simulink model "SimulacaocomVTeCA"  (R2024b)
settings: Solver=VariableStepAuto  StartTime=0.0  StopTime=10  RelTol=1e-3
values from neighbouring files (symbols this model uses):
  AirTemperature = 303    [CodigoVT.m]
  C1 = 1.2801    [CodigoVT.m]
  C2 = 23.99    [CodigoVT.m]
  C3 = 0.52    [CodigoVT.m]
  VelRef = 30    [CodigoVT.m]
undefined symbols (not defined in the file or in its folder): EV, fractalcoef, MTR
libraries: vehdynlibtire x4, slpidlib x2, autolibmappedmotor x2, vrlib x1, mspsensorlib x1, vehdynlibviscommon x1, vehdynlibscenariocommon x1, vehdynlibsuspension x1, vehdynlibsteering x1, vehdynlibdriver x1, autolibshared x1
(part 3 of 3)

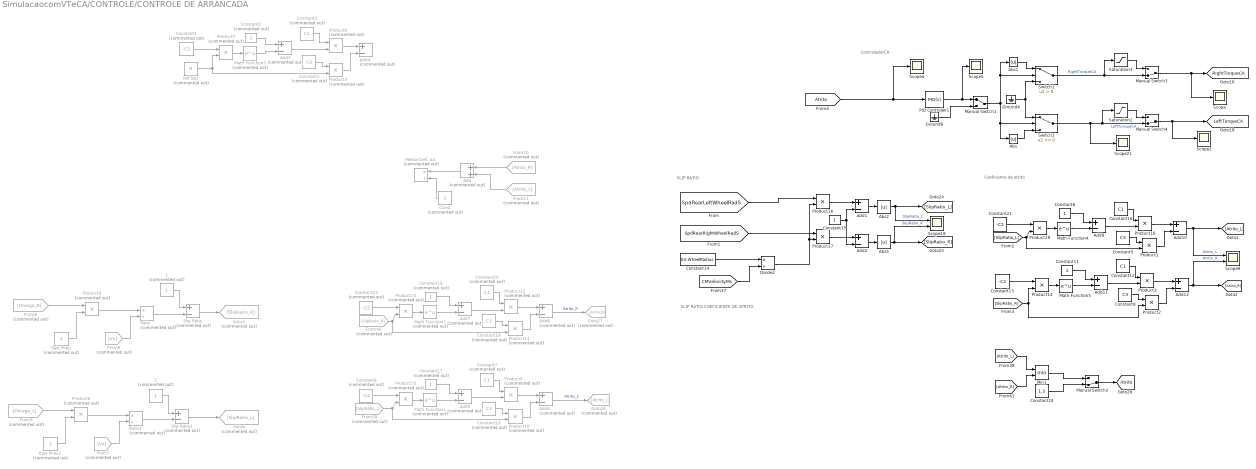
== system SimulacaocomVTeCA/CONTROLE/CONTROLE DE ARRANCADA  ==
  note: ControladorCA
  note: SLIP RATIO
  note: SLIP RATIO
      |
      | COEFICIENTE DE ATRITO
  note: Coeficiente de atrito
  1 : Constant  Commented=on
  2 : Constant  Commented=on
  Abs{,1..2,5} (4 alike) : Abs  SaturateOnIntegerOverflow=off
  Add : Sum  Commented=on
  Add{1..2,9..12} (6 alike) : Sum  Inputs=+-
  Add{3..8} (6 alike) : Sum  Commented=on  Inputs=+-
  Const : Constant  Commented=on  Value=2
  Constant1 : Constant  Commented=on  Value=C3
  Constant10 : Constant  Commented=on  Value=C3
  Constant11 : Constant
  Constant12 : Constant  Value=C1
  Constant13 : Constant  Value=-C2
  Constant14 : Constant  Value=EV.WheelRadius  VectorParams1D=off
  Constant15 : Constant
  Constant16 : Constant  Value=C1
  Constant17 : Constant  Commented=on
  Constant18 : Constant  Commented=on  Value=C3
  Constant19 : Constant  Commented=on
  Constant2 : Constant  Commented=on
  Constant20 : Constant  Commented=on  Value=C1
  Constant21 : Constant  Value=-C2
  Constant23 : Constant  Commented=on  Value=-C2
  Constant24 : Constant  Value=1.3  VectorParams1D=off
  Constant3 : Constant  Commented=on  Value=C1
  Constant4 : Constant  Commented=on  Value=-C2
  Constant5 : Constant  Value=C3
  Constant6 : Constant
  Constant7 : Constant  Commented=on  Value=C1
  Constant8 : Constant  Commented=on  Value=-C2
  Constant9 : Constant  Value=C3
  Divide2 : Product  Inputs=*/
  From10 : From  Commented=on  GotoTag=Atrito_R
  From11 : From  Commented=on  GotoTag=Atrito_L
  From39 : From  Commented=on  GotoTag=SlipRatio_L
  From40 : From  Commented=on  GotoTag=SlipRatio_R
  From6 : From  Commented=on  GotoTag=Vx
  From7 : From  Commented=on  GotoTag=Vx
  From8 : From  Commented=on  GotoTag=Omega_R
  From9 : From  Commented=on  GotoTag=Omega_L
  Goto26 : Goto  Commented=on  GotoTag=Atrito_L
  Goto27 : Goto  Commented=on  GotoTag=Atrito_R
  Goto3 : Goto  Commented=on  GotoTag=SlipRatio_R
  Goto6 : Goto  Commented=on  GotoTag=SlipRatio_L
  Ground4 : Ground
  Ground6 : Ground
  Manual Switch1 : ManualSwitch
  Manual Switch2 : ManualSwitch  CurrentSetting=0
  Manual Switch3 : ManualSwitch  CurrentSetting=0
  Manual Switch4 : ManualSwitch  CurrentSetting=0
  Math Function1 : Math  Commented=on
  Math Function2 : Math  Commented=on
  Math Function3 : Math  Commented=on
  Math Function4 : Math
  Math Function5 : Math
  Min1 : MinMax  Inputs=2
  Média Coef. Ad. : Product  Commented=on  Inputs=*/
  PID Controller1 : slpidlib/PID Controller  Controller=PID  Form=Parallel  TimeDomain=Continuous-time  UseExternalTs=off  SampleTime=-1  IntegratorMethod=Forward Euler  FilterMethod=Forward Euler  ControllerParametersSource=internal  P=1  I=1  UseKiTs=off  D=0  UseExternalDerivativeSource=off  N=100  UseFilter=on  TunerSelectOption=Transfer Function Based (PID Tuner App)  InitialConditionSource=internal  InitialConditionForIntegrator=0  InitialConditionForFilter=0  DifferentiatorICPrevScaledInput=0  ExternalReset=none  TrackingMode=off  Kt=1  LimitOutput=off  SatLimitsSource=internal  UpperSaturationLimit=inf  LowerSaturationLimit=-inf  LinearizeAsGain=on  AntiWindupMode=none  Kb=1  LimitIntegrator=off  UpperIntegratorSaturationLimit=inf  LowerIntegratorSaturationLimit=-inf  POutMin=[]  POutMax=[]  IOutMin=[]  IOutMax=[]  DOutMin=[]  DOutMax=[]  NOutMin=[]  NOutMax=[]  SumOutMin=[]  SumOutMax=[]  SaturationOutMin=[]  SaturationOutMax=[]  PParamMin=[]  PParamMax=[]  IParamMin=[]  IParamMax=[]  DParamMin=[]  DParamMax=[]  NParamMin=[]  NParamMax=[]  KbParamMin=[]  KbParamMax=[]  KtParamMin=[]  KtParamMax=[]  KbOutMin=[]  KbOutMax=[]  KtOutMin=[]  KtOutMax=[]  IntegratorOutMin=[]  IntegratorOutMax=[]  FilterOutMin=[]  FilterOutMax=[]  SumI1OutMin=[]  SumI1OutMax=[]  SumI2OutMin=[]  SumI2OutMax=[]  SumI3OutMin=[]  SumI3OutMax=[]  SumI4OutMin=[]  SumI4OutMax=[]  SumDOutMin=[]  SumDOutMax=[]  DifferentiatorOutMin=[]  DifferentiatorOutMax=[]  FilterDiffOutCoefMin=[]  FilterDiffOutCoefMax=[]  ReciprocalOutMin=[]  ReciprocalOutMax=[]  SumDenOutMin=[]  SumDenOutMax=[]  SumNumOutMin=[]  SumNumOutMax=[]  DivideOutMin=[]  DivideOutMax=[]  UdiffTsProdOutMin=[]  UdiffTsProdOutMax=[]  NTsProdOutMin=[]  NTsProdOutMax=[]  UintegralTsProdOutMin=[]  UintegralTsProdOutMax=[]  UngainTsProdOutMin=[]  UngainTsProdOutMax=[]  ClampingZeroOutDataTypeStr=Inherit: Inherit via back propagation  ClampingZeroOutMin=[]  ClampingZeroOutMax=[]  FilterDenConstantOutDataTypeStr=Inherit: Inherit via back propagation  FilterDenConstantOutMin=[]  FilterDenConstantOutMax=[]  PCopyOutDataTypeStr=Inherit: Inherit via back propagation  PCopyOutMin=[]  PCopyOutMax=[]  NCopyOutDataTypeStr=Inherit: Inherit via back propagation  NCopyOutMin=[]  NCopyOutMax=[]  IntegratorContinuousStateAttributes=''  IntegratorStateMustResolveToSignalObject=off  IntegratorRTWStateStorageClass=Auto  FilterContinuousStateAttributes=''  FilterStateMustResolveToSignalObject=off  FilterRTWStateStorageClass=Auto  ParallelPVariant=InternalParameters  IdealPVariant=Disabled  IVariant=InternalParameters  DVariant=InternalParameters  IntegratorVariant=Continuous  SatVariant=Disabled  AWVariant=Passthrough  PCopyVariant=Disabled  TRVariant=Disabled  FdbkBlocksVariant=Forward  IdealPFdbkVariant=Disabled  SatFdbkVariant=Disabled  DerivativeFilterVariant=ContFilter  NVariant=InternalParameters  NCopyVariant=Disabled  FilterICVariant=InternalICsFilter  IntegratorICVariant=InternalICs  ExternalResetVariant=Disabled  TRSumVariant=Passthrough  SumFdbkVariant=Disabled  SumVariant=Sum_PID  TsampFilterVariant=InternalTs  TsampNgainVariant=Passthrough  TsampIntegralVariant=Disabled_SignalSpec  ExternalSaturationOutDataTypeStr=Inherit: Same as second input  DerivativeSourceVariant=ErrorSignal  PreIntVariant=InternalPreInt
  Product{1..3,14,16..19} (8 alike) : Product
  Product{4..13,15} (11 alike) : Product  Commented=on
  Raio Pneu : Constant  Commented=on  Value=2
  Raio Pneu1 : Constant  Commented=on  Value=2
  Ratio : Product  Commented=on  Inputs=*/
  Ratio1 : Product  Commented=on  Inputs=*/
  Ref Slip : Constant  Commented=on  Value=8
  Saturation2 : Saturate  UpperLimit=11.7  LowerLimit=0
  Saturation3 : Saturate  UpperLimit=11.7  LowerLimit=0
  Scope{,2,4..5,21} (5 alike) : Scope
  Scope18 : Scope  NumInputPorts=2
  Scope9 : Scope  NumInputPorts=2
  Slip Ratio : Sum  Commented=on  Inputs=+-
  Slip Ratio1 : Sum  Commented=on  Inputs=+-
  Switch1 : Switch  Criteria=u2 > Threshold  SaturateOnIntegerOverflow=off  InputSameDT=off
  Switch2 : Switch  SaturateOnIntegerOverflow=off  InputSameDT=off
  tag scope: Atrito=global, LeftTorqueCA=global, RightTorqueCA=global
  wires:
  Constant10/1 -> Product10/1
  Constant23/1 -> Product13/1
  Constant19/1 -> Add7/1
  Manual Switch3/1 -> Scope/1, [RightTorqueCA]
  [Atrito] -> Scope4/1, PID Controller1/1
  Math Function2/1 -> Add7/2
  2/1 -> Slip Ratio1/1
  Product8/1 -> Ratio1/1
  Add/1 -> Média Coef. Ad./1
  Product4/1 -> Ratio/1
  Manual Switch4/1 -> Scope2/1, [LeftTorqueCA]
  Math Function1/1 -> Add5/2
  Switch1/1 -> Saturation3/1, Manual Switch3/2  "RightTorqueCA"
  From40/1 -> Product11/2, Product13/2
  Math Function3/1 -> Add3/2
  Ref Slip/1 -> Product7/2, Product5/2
  Product6/1 -> Add4/1
  Manual Switch1/1 -> Abs/1, Switch2/2, Abs1/1, Switch1/2
  PID Controller1/1 -> Scope5/1, Manual Switch1/1
  Product13/1 -> Math Function2/1
  Product12/1 -> Add8/1
  Saturation3/1 -> Manual Switch3/1
  From11/1 -> Add/2
  Constant17/1 -> Add5/1
  Saturation2/1 -> Manual Switch4/1
  Slip Ratio1/1 -> Goto6/1
  From8/1 -> Product4/1
  Constant3/1 -> Product6/1
  Ground4/1 -> Switch1/3, Switch2/1
  From6/1 -> Ratio/2
  Ratio/1 -> Slip Ratio/2
  Constant18/1 -> Product11/1
  Constant20/1 -> Product12/1
  Ratio1/1 -> Slip Ratio1/2
  From9/1 -> Product8/1
  Add5/1 -> Product9/2
  Add6/1 -> Goto26/1  "Atrito_L"
  Product10/1 -> Add6/2
  Constant2/1 -> Add3/1
  Switch2/1 -> Saturation2/1, Manual Switch4/2, Scope21/1  "LeftTorqueCA"
  Add8/1 -> Goto27/1  "Atrito_R"
  From10/1 -> Add/1
  Const/1 -> Média Coef. Ad./2
  Raio Pneu1/1 -> Product8/2
  Product5/1 -> Add4/2
  Constant1/1 -> Product5/1
  Add3/1 -> Product6/2
  Product7/1 -> Math Function3/1
  Product9/1 -> Add6/1
  Abs/1 -> Switch2/3
  Raio Pneu/1 -> Product4/2
  Constant7/1 -> Product9/1
  From39/1 -> Product10/2, Product15/2
  1/1 -> Slip Ratio/1
  Constant4/1 -> Product7/1
  Slip Ratio/1 -> Goto3/1
  From7/1 -> Ratio1/2
  Product15/1 -> Math Function1/1
  Ground6/1 -> Manual Switch1/2
  Add7/1 -> Product12/2
  Constant8/1 -> Product15/1
  Abs1/1 -> Switch1/1
  Product11/1 -> Add8/2
  [CMVelocityMs] -> Divide2/2
  Manual Switch2/1 -> [Atrito]
  Min1/1 -> Manual Switch2/1
  Constant24/1 -> Manual Switch2/2
  Add9/1 -> Product18/2
  [Atrito_L] -> Min1/1
  Math Function5/1 -> Add11/2
  Constant15/1 -> Add1/2, Add2/2
  Constant11/1 -> Add11/1
  Constant16/1 -> Product18/1
  Product1/1 -> Add10/2
  Constant9/1 -> Product2/1
  Math Function4/1 -> Add9/2
  Constant5/1 -> Product1/1
  Constant6/1 -> Add9/1
  Constant21/1 -> Product19/1
  Add10/1 -> Scope9/1, [Atrito_L]  "Atrito_L"
  Product19/1 -> Math Function4/1
  [SpdRearLeftWheelRadS] -> Product16/1
  Product16/1 -> Add1/1
  Product2/1 -> Add12/2
  [SpdRearRightWheelRadS] -> Product17/1
  Add11/1 -> Product3/2
  Add1/1 -> Abs2/1
  Abs2/1 -> Scope18/1, [SlipRatio_L]  "SlipRatio_L"
  Constant12/1 -> Product3/1
  Product3/1 -> Add12/1
  Product17/1 -> Add2/1
  [SlipRatio_R] -> Product14/2, Product2/2
  Constant14/1 -> Divide2/1
  Product14/1 -> Math Function5/1
  Divide2/1 -> Product16/2, Product17/2
  Abs5/1 -> Scope18/2, [SlipRatio_R]  "SlipRatio_R"
  Add12/1 -> Scope9/2, [Atrito_R]  "Atrito_R"
  Product18/1 -> Add10/1
  [Atrito_R] -> Min1/2
  [SlipRatio_L] -> Product1/2, Product19/2
  Add2/1 -> Abs5/1
  Constant13/1 -> Product14/1

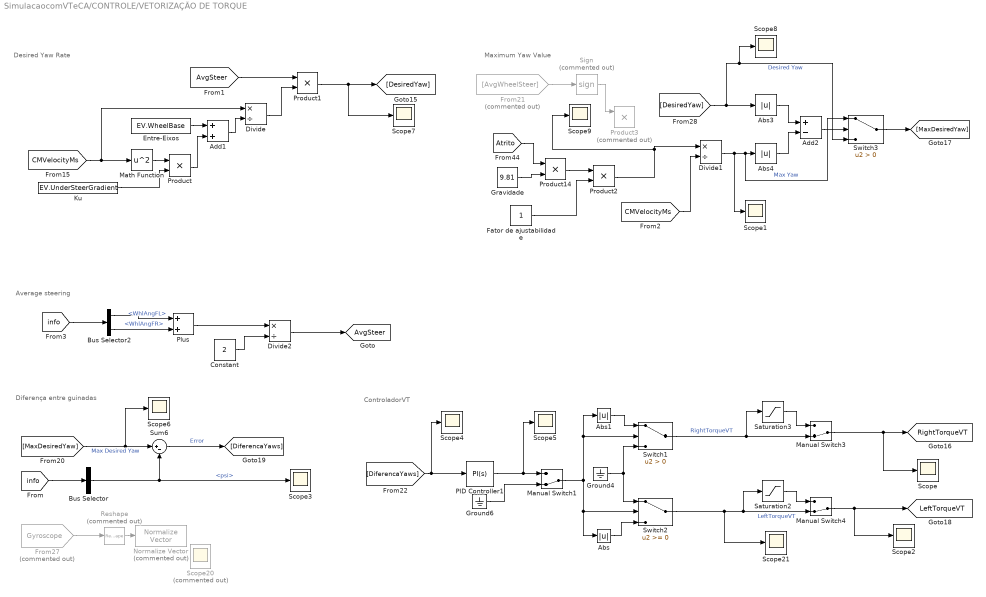
== system SimulacaocomVTeCA/CONTROLE/VETORIZAÇÃO DE TORQUE  ==
  note: Average steering
  note: Desired Yaw Rate
  note: Maximum Yaw Value
  note: Diferença entre guinadas
  note: ControladorVT
  Abs{,1,3..4} (4 alike) : Abs  SaturateOnIntegerOverflow=off
  Add1 : Sum
  Add2 : Sum  Inputs=+-
  Bus Selector : BusSelector  OutputSignals=InertFrm.Cg.Ang.psi
  Bus Selector2 : BusSelector  OutputSignals=BdyFrm.FrntAxl.Steer.WhlAngFL,BdyFrm.FrntAxl.Steer.WhlAngFR
  Constant : Constant  Value=2
  Divide : Product  Inputs=*/
  Divide1 : Product  Inputs=*/
  Divide2 : Product  Inputs=*/
  Entre-Eixos : Constant  Value=EV.WheelBase
  Fator de ajustabilidade : Constant
  From21 : From  Commented=on  GotoTag=AvgWheelSteer
  From27 : From  Commented=on  GotoTag=Gyroscope  TagVisibility=global
  Gravidade : Constant  Value=9.81
  Ground4 : Ground
  Ground6 : Ground
  Ku : Constant  Value=EV.UnderSteerGradient
  Manual Switch1 : ManualSwitch  CurrentSetting=0
  Manual Switch3 : ManualSwitch  CurrentSetting=0
  Manual Switch4 : ManualSwitch  CurrentSetting=0
  Math Function : Math  Operator=square
  Normalize Vector : vrlib/Utilities/Normalize Vector  Commented=on  maxzero=0
  PID Controller1 : slpidlib/PID Controller  Controller=PI  Form=Parallel  TimeDomain=Continuous-time  UseExternalTs=off  SampleTime=-1  IntegratorMethod=Forward Euler  FilterMethod=Forward Euler  ControllerParametersSource=internal  P=0  I=-1  UseKiTs=off  D=-1.04450033164761  UseExternalDerivativeSource=off  N=21.9051072982779  UseFilter=on  TunerSelectOption=Transfer Function Based (PID Tuner App)  InitialConditionSource=internal  InitialConditionForIntegrator=0  InitialConditionForFilter=0  DifferentiatorICPrevScaledInput=0  ExternalReset=none  TrackingMode=off  Kt=1  LimitOutput=off  SatLimitsSource=internal  UpperSaturationLimit=inf  LowerSaturationLimit=-inf  LinearizeAsGain=on  AntiWindupMode=none  Kb=1  LimitIntegrator=off  UpperIntegratorSaturationLimit=inf  LowerIntegratorSaturationLimit=-inf  POutMin=[]  POutMax=[]  IOutMin=[]  IOutMax=[]  DOutMin=[]  DOutMax=[]  NOutMin=[]  NOutMax=[]  SumOutMin=[]  SumOutMax=[]  SaturationOutMin=[]  SaturationOutMax=[]  PParamMin=[]  PParamMax=[]  IParamMin=[]  IParamMax=[]  DParamMin=[]  DParamMax=[]  NParamMin=[]  NParamMax=[]  KbParamMin=[]  KbParamMax=[]  KtParamMin=[]  KtParamMax=[]  KbOutMin=[]  KbOutMax=[]  KtOutMin=[]  KtOutMax=[]  IntegratorOutMin=[]  IntegratorOutMax=[]  FilterOutMin=[]  FilterOutMax=[]  SumI1OutMin=[]  SumI1OutMax=[]  SumI2OutMin=[]  SumI2OutMax=[]  SumI3OutMin=[]  SumI3OutMax=[]  SumI4OutMin=[]  SumI4OutMax=[]  SumDOutMin=[]  SumDOutMax=[]  DifferentiatorOutMin=[]  DifferentiatorOutMax=[]  FilterDiffOutCoefMin=[]  FilterDiffOutCoefMax=[]  ReciprocalOutMin=[]  ReciprocalOutMax=[]  SumDenOutMin=[]  SumDenOutMax=[]  SumNumOutMin=[]  SumNumOutMax=[]  DivideOutMin=[]  DivideOutMax=[]  UdiffTsProdOutMin=[]  UdiffTsProdOutMax=[]  NTsProdOutMin=[]  NTsProdOutMax=[]  UintegralTsProdOutMin=[]  UintegralTsProdOutMax=[]  UngainTsProdOutMin=[]  UngainTsProdOutMax=[]  ClampingZeroOutDataTypeStr=Inherit: Inherit via back propagation  ClampingZeroOutMin=[]  ClampingZeroOutMax=[]  FilterDenConstantOutDataTypeStr=Inherit: Inherit via back propagation  FilterDenConstantOutMin=[]  FilterDenConstantOutMax=[]  PCopyOutDataTypeStr=Inherit: Inherit via back propagation  PCopyOutMin=[]  PCopyOutMax=[]  NCopyOutDataTypeStr=Inherit: Inherit via back propagation  NCopyOutMin=[]  NCopyOutMax=[]  IntegratorContinuousStateAttributes=''  IntegratorStateMustResolveToSignalObject=off  IntegratorRTWStateStorageClass=Auto  FilterContinuousStateAttributes=''  FilterStateMustResolveToSignalObject=off  FilterRTWStateStorageClass=Auto  ParallelPVariant=InternalParameters  IdealPVariant=Disabled  IVariant=InternalParameters  DVariant=Disabled  IntegratorVariant=Continuous  SatVariant=Disabled  AWVariant=Passthrough  PCopyVariant=Disabled  TRVariant=Disabled  FdbkBlocksVariant=Forward  IdealPFdbkVariant=Disabled  SatFdbkVariant=Disabled  DerivativeFilterVariant=Disabled  NVariant=Disabled  NCopyVariant=Disabled_SignalSpec  FilterICVariant=Disabled  IntegratorICVariant=InternalICs  ExternalResetVariant=Disabled  TRSumVariant=Passthrough  SumFdbkVariant=Disabled  SumVariant=Sum_PI  TsampFilterVariant=InternalTs  TsampNgainVariant=Passthrough  TsampIntegralVariant=Disabled_SignalSpec  ExternalSaturationOutDataTypeStr=Inherit: Same as second input  DerivativeSourceVariant=Disabled  PreIntVariant=InternalPreInt
  Plus : Sum
  Product{,1..2,14} (4 alike) : Product
  Product3 : Product  Commented=on
  Reshape : Reshape  Commented=on
  Saturation2 : Saturate  UpperLimit=11.7  LowerLimit=0
  Saturation3 : Saturate  UpperLimit=11.7  LowerLimit=0
  Scope{,1..9,21} (11 alike) : Scope
  Scope20 : Scope  Commented=on
  Sign : Signum  Commented=on
  Sum6 : Sum  Inputs=|+-
  Switch1 : Switch  Criteria=u2 > Threshold  SaturateOnIntegerOverflow=off  InputSameDT=off
  Switch2 : Switch  SaturateOnIntegerOverflow=off  InputSameDT=off
  Switch3 : Switch  Criteria=u2 > Threshold  SaturateOnIntegerOverflow=off  InputSameDT=off
  tag scope: AvgSteer=global, LeftTorqueVT=global, RightTorqueVT=global
  wires:
  Product1/1 -> Scope7/1, [DesiredYaw]
  Math Function/1 -> Product/1
  Entre-Eixos/1 -> Add1/1
  Ku/1 -> Product/2
  Product/1 -> Add1/2
  Add1/1 -> Divide/2
  [CMVelocityMs] -> Divide/1, Math Function/1
  From21/1 -> Sign/1
  [Atrito] -> Product14/1
  Add2/1 -> Switch3/2
  [DesiredYaw] -> Abs3/1, Scope8/1, Switch3/3  "Desired Yaw"
  Product14/1 -> Product2/1
  Divide1/1 -> Scope1/1, Switch3/1, Abs4/1  "Max Yaw"
  Sign/1 -> Product3/1
  Abs4/1 -> Add2/2
  Fator de ajustabilidade/1 -> Product2/2
  Abs3/1 -> Add2/1
  Switch3/1 -> [MaxDesiredYaw]
  Gravidade/1 -> Product14/2
  [MaxDesiredYaw] -> Scope6/1, Sum6/1  "Max Desired Yaw"
  Sum6/1 -> [DiferencaYaws]  "Error"
  Manual Switch3/1 -> Scope/1, [RightTorqueVT]
  Abs/1 -> Switch2/3
  Ground4/1 -> Switch1/3, Switch2/1
  PID Controller1/1 -> Scope5/1, Manual Switch1/1
  Saturation3/1 -> Manual Switch3/1
  Switch1/1 -> Saturation3/1, Manual Switch3/2  "RightTorqueVT"
  Abs1/1 -> Switch1/1
  Manual Switch1/1 -> Abs/1, Switch2/2, Abs1/1, Switch1/2
  Ground6/1 -> Manual Switch1/2
  Manual Switch4/1 -> Scope2/1, [LeftTorqueVT]
  Switch2/1 -> Saturation2/1, Manual Switch4/2, Scope21/1  "LeftTorqueVT"
  Saturation2/1 -> Manual Switch4/1
  [DiferencaYaws] -> Scope4/1, PID Controller1/1
  From27/1 -> Reshape/1
  Reshape/1 -> Normalize Vector/1
  [info] -> Bus Selector/1
  Bus Selector/1 -> Scope3/1, Sum6/2  "<psi>"
  Product2/1 -> Scope9/1, Divide1/1
  [CMVelocityMs] -> Divide1/2
  [info] -> Bus Selector2/1
  Bus Selector2/2 -> Plus/2  "<WhlAngFR>"
  Bus Selector2/1 -> Plus/1  "<WhlAngFL>"
  Plus/1 -> Divide2/1
  Constant/1 -> Divide2/2
  Divide2/1 -> [AvgSteer]
  Divide/1 -> Product1/2
  [AvgSteer] -> Product1/1

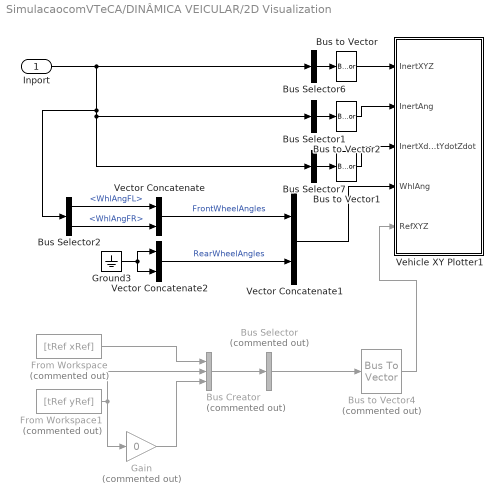
== system SimulacaocomVTeCA/DINÂMICA VEICULAR/2D Visualization ==
  Inport : Inport
  Bus Creator : BusCreator  Commented=on  Inputs=3
  Bus Selector : BusSelector  Commented=on  OutputSignals=signal1,signal2,signal3  OutputAsBus=on
  Bus Selector1 : BusSelector  OutputSignals=InertFrm.Cg.Ang.phi,InertFrm.Cg.Ang.theta,InertFrm.Cg.Ang.psi  OutputAsBus=on
  Bus Selector2 : BusSelector  OutputSignals=BdyFrm.FrntAxl.Steer.WhlAngFL,BdyFrm.FrntAxl.Steer.WhlAngFR
  Bus Selector6 : BusSelector  OutputSignals=InertFrm.Geom.Disp.X,InertFrm.Geom.Disp.Y,InertFrm.Geom.Disp.Z  OutputAsBus=on
  Bus Selector7 : BusSelector  OutputSignals=InertFrm.Geom.Vel.Xdot,InertFrm.Geom.Vel.Ydot,InertFrm.Geom.Vel.Zdot  OutputAsBus=on
  Bus to Vector : BusToVector
  Bus to Vector1 : BusToVector
  Bus to Vector2 : BusToVector
  Bus to Vector4 : BusToVector  Commented=on
  From Workspace : FromWorkspace  Commented=on  VariableName=[tRef xRef]
  From Workspace1 : FromWorkspace  Commented=on  VariableName=[tRef yRef]
  Gain : Gain  Commented=on  Gain=0
  Ground3 : Ground
  Vector Concatenate : Concatenate
  Vector Concatenate1 : Concatenate
  Vector Concatenate2 : Concatenate
  Vehicle XY Plotter1 : Subsystem  mask(Vehicle XY Plotter){extRef=on, extStats=off, extTireF=off, a=2, b=2, w=2, figBorder=10, bufferSize=1024, velNorm=5, tireFNorm=1000, pltDT=0.2}
      mask prompts: extRef "Plot path reference, extRef"; extStats "Display speed, RPM and Gear"; extTireF "Display tire forces"; a "Distance to front axle from CG, a [m]:"; b "Distance to rear axle from CG, b [m]:"; w "Track width, w [m]:"; figBorder "Distance to figure borders, figBorder [m]:"; bufferSize "Path buffer sampe size, bufferSize []:"; velNorm "Velocity vector scaling, velNorm [m*s/m]:"; tireFNorm "Tire force vector scaling, tireFNorm [m/N]:"; pltDT "Plot update rate, pltDT [s]:"
      mask help:
      | This block will display a MATLAB figure which indicates the vehicle path, current position and heading velocity.
      | An optional path reference is also provided.
      mask init:
      | block = gcb;
      | if autoblkschecksimstopped(block)
      |     ParamNames = {'extRef';'extStats';'extTireF';'extTireF'};
      |     PortNames = {'RefXYZ';'Stats';'TireFx';'TireFy'};
      |     for idx=1:length(PortNames)
      |         InportOption  = {'built-in/Ground', [PortNames{idx}, ' Ground'];...
      |             'built-in/Inport',PortNames{idx}};
      |         if ~strcmp(get_param(block,ParamNames{idx}),'on')
      |             NewBlkHdl = autoblksreplaceblock(block, InportOption, 1);
      |             set_param(NewBlkHdl, 'ShowName', 'off');
      |         else
      |             autoblksreplaceblock(block, InportOption, 2);
      |         end
      |     end
      |     InportNames = {'InertXYZ';'InertAng';'InertXdotYdotZdot';'WhlAng';'RefXYZ';'Stats';'TireFx';'TireFy'};
      |     FoundNames = get_param(find_system(block, 'LookUnderMasks', 'all', 'SearchDepth', 1, 'FollowLinks', 'on', 'BlockType', 'Inport'), 'Name');
      |     [~,PortI] = intersect(InportNames, FoundNames);
      |     PortI = sort(PortI);
      |     for idx = 1:length(PortI)
      |         set_param([block, '/', InportNames{PortI(idx)}], 'Port', num2str(idx));
      |     end
      | end
      mask TypeOptions a: Vehicle XY Plotter/a
      mask TypeOptions b: Vehicle XY Plotter/b
      mask TypeOptions w: Vehicle XY Plotter/w
      mask TypeOptions figBorder: Vehicle XY Plotter/figBorder
      mask TypeOptions bufferSize: Vehicle XY Plotter/bufferSize
      mask TypeOptions velNorm: Vehicle XY Plotter/velNorm
      mask TypeOptions tireFNorm: Vehicle XY Plotter/tireFNorm
      mask DialogControl Container3 Prompt: Plot and Display Options
  wires:
  Vector Concatenate1/1 -> Vehicle XY Plotter1/4(WhlAng)
  Ground3/1 -> Vector Concatenate2/1, Vector Concatenate2/2
  Bus Selector6/1 -> Bus to Vector/1
  Vector Concatenate/1 -> Vector Concatenate1/1  "FrontWheelAngles"
  Vector Concatenate2/1 -> Vector Concatenate1/2  "RearWheelAngles"
  Bus Selector7/1 -> Bus to Vector1/1
  Bus to Vector1/1 -> Vehicle XY Plotter1/3(InertXdotYdotZdot)
  Bus to Vector/1 -> Vehicle XY Plotter1/1(InertXYZ)
  Bus to Vector2/1 -> Vehicle XY Plotter1/2(InertAng)
  Bus Selector1/1 -> Bus to Vector2/1
  Inport/1 -> Bus Selector2/1, Bus Selector7/1, Bus Selector1/1, Bus Selector6/1
  Bus to Vector4/1 -> Vehicle XY Plotter1/5(RefXYZ)
  Bus Selector/1 -> Bus to Vector4/1
  From Workspace1/1 -> Gain/1, Bus Creator/2
  Gain/1 -> Bus Creator/3
  From Workspace/1 -> Bus Creator/1
  Bus Creator/1 -> Bus Selector/1
  Bus Selector2/1 -> Vector Concatenate/1  "<WhlAngFL>"
  Bus Selector2/2 -> Vector Concatenate/2  "<WhlAngFR>"

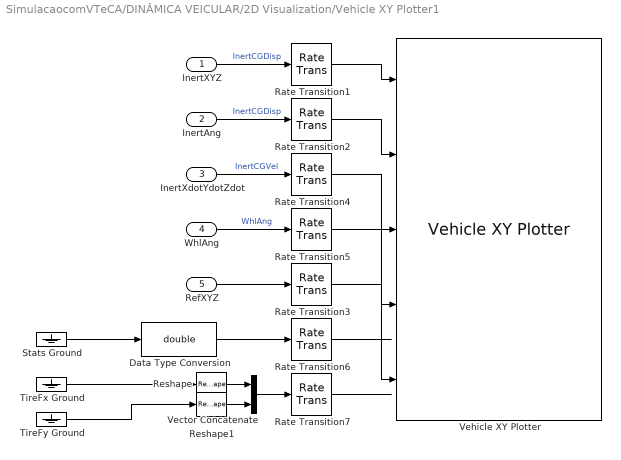
== system SimulacaocomVTeCA/DINÂMICA VEICULAR/2D Visualization/Vehicle XY Plotter1 ==
  InertXYZ : Inport
  InertAng : Inport  Port=2
  InertXdotYdotZdot : Inport  Port=3
  WhlAng : Inport  Port=4
  RefXYZ : Inport  Port=5
  Data Type Conversion : DataTypeConversion  OutDataTypeStr=double  SaturateOnIntegerOverflow=off  RndMeth=Floor
  Rate Transition{1..7} (7 alike) : RateTransition  Deterministic=off  OutPortSampleTime=pltDT
  Reshape : Reshape  OutputDimensionality=Row vector (2-D)
  Reshape1 : Reshape  OutputDimensionality=Row vector (2-D)
  Stats Ground : Ground
  TireFx Ground : Ground
  TireFy Ground : Ground
  Vector Concatenate : Concatenate  Mode=Multidimensional array
  Vehicle XY Plotter : vehdynlibviscommon/Vehicle XY Plotter  w=w  a=a  b=b  figBorder=figBorder  bufferSize=bufferSize  extStats=off  extTireF=off
  wires:
  Vector Concatenate/1 -> Rate Transition7/1
  Reshape1/1 -> Vector Concatenate/2
  Reshape/1 -> Vector Concatenate/1
  RefXYZ/1 -> Rate Transition3/1
  Rate Transition7/1 -> ?
  Data Type Conversion/1 -> Rate Transition6/1
  Rate Transition6/1 -> ?
  Rate Transition5/1 -> Vehicle XY Plotter/4
  Rate Transition4/1 -> Vehicle XY Plotter/3
  Rate Transition2/1 -> Vehicle XY Plotter/2
  Rate Transition1/1 -> Vehicle XY Plotter/1
  Rate Transition3/1 -> Vehicle XY Plotter/5
  WhlAng/1 -> Rate Transition5/1  "WhlAng"
  InertXYZ/1 -> Rate Transition1/1  "InertCGDisp"
  InertXdotYdotZdot/1 -> Rate Transition4/1  "InertCGVel"
  InertAng/1 -> Rate Transition2/1  "InertCGDisp"
  Stats Ground/1 -> Data Type Conversion/1
  TireFx Ground/1 -> Reshape/1
  TireFy Ground/1 -> Reshape1/1
